simulink model "oscillator"  (R2023b)
settings: Solver=FixedStepAuto  StartTime=0.0  StopTime=15  FixedStep=1e-5  RelTol=1e-3
InitFcn:
  | a=1;
  | %kp=0;
  | %ki=0.01;
  | %h=0.1;
values from neighbouring files (symbols this model uses):
  h = 1    [regions_kpki_Oscillator.m]    (also in responsesOscillator.m = hh(j))
  ki = zeros(length(l),length(kp))    [regions_kpki_Oscillator.m]    (also in responsesOscillator.m = kii(j))
  kp = 5    [regions_hki_Oscillator.m]    (also in regions_kpki_Oscillator.m = linspace(-1000,1000,2); responsesOscillator.m = kpp(j))
settings Model: Creator=JULIAN  LastModifiedBy=jhern
settings OptimizationCC: ReuseModelBlockBuffer=off
settings DebuggingCC: UnconnectedInputMsg=warning  UnconnectedOutputMsg=warning  UnconnectedLineMsg=warning
settings ModelReferenceCC: EnableRefExpFcnMdlSchedulingChecks=on
settings RTWCC: DLArmComputeVersion=19.05

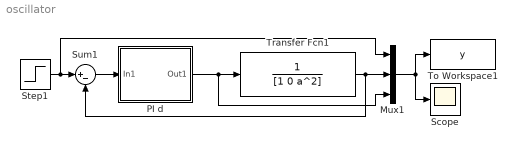
== system oscillator ==
  Mux1 : Mux  Inputs=3
  PI d : Subsystem
  Scope : Scope
  Step1 : Step  Time=0  Before=1  SampleTime=0
  Sum1 : Sum  Inputs=|+-
  To Workspace1 : ToWorkspace  VariableName=y  SampleTime=-1
  Transfer Fcn1 : TransferFcn  Denominator=[1 0 a^2]
  wires:
  Mux1/1 -> To Workspace1/1, Scope/1
  Step1/1 -> Mux1/1, Sum1/1
  Transfer Fcn1/1 -> Mux1/2, Sum1/2
  PI d/1(Out1) -> Transfer Fcn1/1, Mux1/3
  Sum1/1 -> PI d/1(In1)

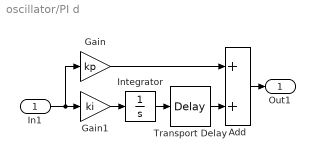
== system oscillator/PI d ==
  In1 : Inport
  Add : Sum
  Gain : Gain  Gain=kp
  Gain1 : Gain  Gain=ki
  Integrator : Integrator
  Transport Delay : TransportDelay  DelayTime=h
  Out1 : Outport
  wires:
  Gain/1 -> Add/1
  In1/1 -> Gain/1, Gain1/1
  Gain1/1 -> Integrator/1
  Add/1 -> Out1/1
  Transport Delay/1 -> Add/2
  Integrator/1 -> Transport Delay/1
